simulink model "Forward_Converter_Using_Goto_From"  (R2023a)
settings: Solver=VariableStepAuto  StartTime=0.0  StopTime=2  RelTol=1e-3
libraries: spsSeriesRLCBranchLib x3, spsVoltageMeasurementLib x3, spsDiodeLib x2, spsDCVoltageSourceLib x1, spsLinearTransformerLib x1, spsMosfetLib x1, spsCurrentMeasurementLib x1, sps_lib x1
settings Model: Creator=vande  LastModifiedBy=vande

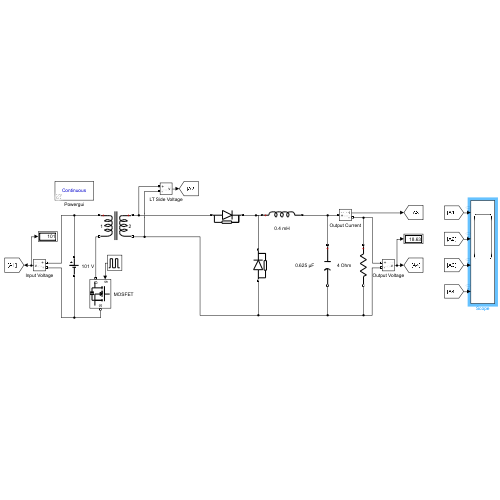
[thumbnail: Simulink's stored preview of the top-level diagram]
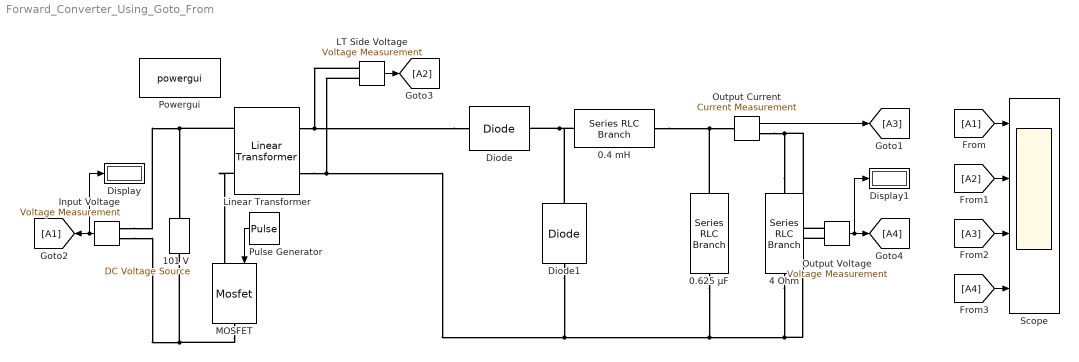
== system Forward_Converter_Using_Goto_From ==
  0.4 mH : spsSeriesRLCBranchLib/Series RLC Branch  LConnTagsString=__new0  RConnTagsString=__new0  BranchType=L  Resistance=1  Inductance=0.4e-3  SetiL0=off  InitialCurrent=0  Capacitance=1e-6  Setx0=off  InitialVoltage=0  Measurements=None
  "0.625 µF " : spsSeriesRLCBranchLib/Series RLC Branch  LConnTagsString=__new0  RConnTagsString=__new0  BranchType=C  Resistance=1  Inductance=1e-3  SetiL0=off  InitialCurrent=0  Capacitance=0.625e-6  Setx0=off  InitialVoltage=0  Measurements=None
  101 V : spsDCVoltageSourceLib/DC Voltage Source  Amplitude=101  Measurements=None
  4 Ohm : spsSeriesRLCBranchLib/Series RLC Branch  LConnTagsString=__new0  RConnTagsString=__new0  BranchType=R  Resistance=4  Inductance=1e-3  SetiL0=off  InitialCurrent=0  Capacitance=1e-6  Setx0=off  InitialVoltage=0  Measurements=None
  Diode : spsDiodeLib/Diode  Ron=0.001  Lon=0  Vf=0.8  IC=0  UseSnubber=0  Rs=500  Cs=250e-9  Measurements=off
  Diode1 : spsDiodeLib/Diode  Ron=0.001  Lon=0  Vf=0.8  IC=0  UseSnubber=0  Rs=500  Cs=250e-9  Measurements=off
  Display : Display
  Display1 : Display
  Input Voltage : spsVoltageMeasurementLib/Voltage Measurement  PhasorSimulation=off  OutputType=Complex  PSBequivalent=0
  LT Side Voltage : spsVoltageMeasurementLib/Voltage Measurement  PhasorSimulation=off  OutputType=Complex  PSBequivalent=0
  Linear Transformer : spsLinearTransformerLib/Linear Transformer  UNITS=SI  NominalPower="[100  50000 ]"  winding1=[101 0 0]  winding2=[40 0 0]  ThreeWindings=off  winding3=[3.15e+05 3.969e+06 505.35]  RmLm=[5.4022e+12 1.7196e+07]  Measurements=None  DataType=on
  MOSFET : spsMosfetLib/Mosfet  Ron=0.1  Lon=0  Rd=0.01  Vfd=0  IC=0  Rs=1e5  Cs=inf  Measurements=off
  Output Current : spsCurrentMeasurementLib/Current Measurement  PhasorSimulation=off  OutputType=Complex  PSBequivalent=0
  Output Voltage : spsVoltageMeasurementLib/Voltage Measurement  PhasorSimulation=off  OutputType=Complex  PSBequivalent=0
  Powergui : sps_lib/powergui  Priority=1  SimulationMode=Continuous  SampleTime=50e-6  frequency=60  Iterations=50  frequencyindice=0  Pbase=100e6  ErrMax=1e-4  UnitsV=kV  UnitsW=MW  buscounter=0  FunctionMessages=off  echomessages=off  EnableUseOfTLC=off  CurrentSourceSwitches=off  DisableSnubberDevices=off  DisableRonSwitches=off  DisableVfSwitches=off  DisplayEquations=off  AutomaticDiscreteSolvers=off  SolverType=Tustin/Backward Euler (TBE)  Interpol=off  ExternalGateDelay=off  methode=off  Ts=100  x0status=blocks  SPID=on  SwTol=0  HookPort=off  NonlinearTolerance=1e-4  nMaxIteration=100  ContinueOnMaxIteration=off  RestoreLinks=warning  ResistiveCurrentMeasurement=off  Frange=[0:2:500]  Ylog=off  Xlog=on  ShowGrid=off  save=off  variable=ZData  structure=0  ZoomFFT=off  StartTime=0.0  cycles=1  DisplayStyle=1  fundamental=60  FreqAxis=off  MaxFrequency=1000  frequencyindicesteady=1  RmsSteady=1  display=off
  Pulse Generator : DiscretePulseGenerator  PulseType=Time based  Amplitude=10  Period=0.00002  PulseWidth=50
  Scope : Scope  NumInputPorts=4
  wires:
  Output Current/1 -> [A3]
  Output Voltage/1 -> Display1/1, [A4]
  Pulse Generator/1 -> MOSFET/1
  LT Side Voltage/1 -> [A2]
  Input Voltage/1 -> Display/1, [A1]
  [A1] -> Scope/1
  [A3] -> Scope/3
  [A4] -> Scope/4
  [A2] -> Scope/2
  connections:
  4 Ohm/LConn1 -- Output Current/RConn1 -- Output Voltage/LConn1
  Linear Transformer/RConn2 -- LT Side Voltage/LConn2 -- Diode1/LConn1 -- 4 Ohm/RConn1 -- Output Voltage/LConn2 -- "0.625 µF "/RConn1
  "0.625 µF "/LConn1 -- Output Current/LConn1 -- 0.4 mH/RConn1
  MOSFET/RConn1 -- Input Voltage/LConn2 -- 101 V/LConn1
  Diode/LConn1 -- Linear Transformer/RConn1 -- LT Side Voltage/LConn1
  Input Voltage/LConn1 -- Linear Transformer/LConn1 -- 101 V/RConn1
  Linear Transformer/LConn2 -- MOSFET/LConn1
  Diode/RConn1 -- Diode1/RConn1 -- 0.4 mH/LConn1
